simulink model "HW4Prob2"  (R2021a)
settings: Solver=VariableStepAuto  StartTime=0.0  StopTime=10.0  RelTol=1e-3
model workspace (MAT data in the model file):
  L = 1
  theta_dot = 1
  v = 1
  vL = 1
  vR = 1
  w = 1
undefined symbols (not defined in the file): IC, kh, kv, p
settings Model: Creator=Jacob  LastModifiedBy=Jacob

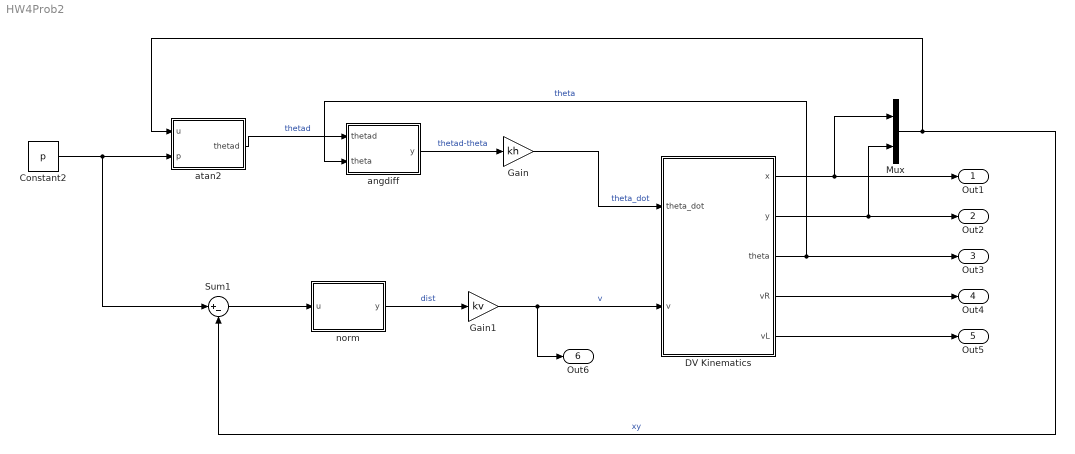
== system HW4Prob2 ==
  Constant2 : Constant  Value=p  VectorParams1D=off
  DV Kinematics : Subsystem
  Gain : Gain  Gain=kh
  Gain1 : Gain  Gain=kv
  Mux : Mux  Inputs=2
  Sum1 : Sum  Inputs=|+-
  angdiff : MATLAB Function  TreatAsAtomicUnit=on
  atan2 : MATLAB Function  TreatAsAtomicUnit=on
  norm : MATLAB Function  TreatAsAtomicUnit=on
  Out1 : Outport  SignalName=x
  Out2 : Outport  Port=2  SignalName=y
  Out3 : Outport  Port=3  SignalName=theta
  Out4 : Outport  Port=4  SignalName=vR
  Out5 : Outport  Port=5  SignalName=vL
  Out6 : Outport  Port=6  SignalName=v
  wires:
  Gain/1 -> DV Kinematics/1(theta_dot)  "theta_dot"
  Gain1/1 -> Out6/1, DV Kinematics/2(v)  "v"
  DV Kinematics/1(x) -> Mux/1, Out1/1
  DV Kinematics/2(y) -> Mux/2, Out2/1
  DV Kinematics/3(theta) -> Out3/1, angdiff/2(theta)  "theta"
  DV Kinematics/4(vR) -> Out4/1
  DV Kinematics/5(vL) -> Out5/1
  Mux/1 -> atan2/1(u), Sum1/2  "xy"
  Constant2/1 -> Sum1/1, atan2/2(p)
  Sum1/1 -> norm/1(u)
  norm/1(y) -> Gain1/1  "dist"
  angdiff/1(y) -> Gain/1  "thetad-theta"
  atan2/1(thetad) -> angdiff/1(thetad)  "thetad"

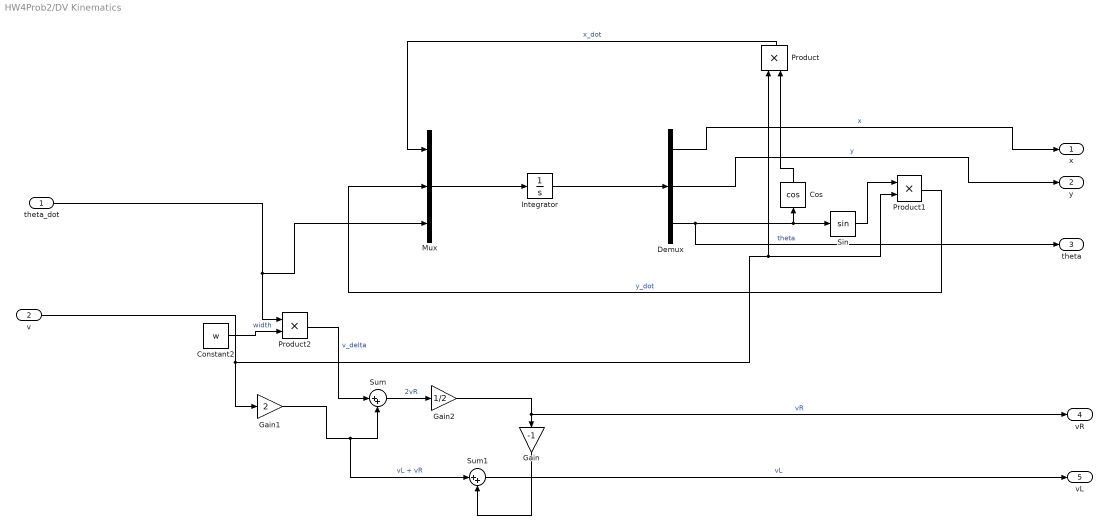
== system HW4Prob2/DV Kinematics ==
  theta_dot : Inport
  v : Inport  Port=2
  Constant2 : Constant  Value=w
  Cos : Trigonometry  Operator=cos
  Demux : Demux  Outputs=3
  Gain : Gain  Gain=-1
  Gain1 : Gain  Gain=2
  Gain2 : Gain  Gain=1/2
  Integrator : Integrator  InitialCondition=IC
  Mux : Mux  Inputs=3
  Product : Product
  Product1 : Product
  Product2 : Product
  Sin : Trigonometry
  Sum : Sum  Inputs=|++
  Sum1 : Sum  Inputs=|++
  x : Outport
  y : Outport  Port=2
  theta : Outport  Port=3
  vR : Outport  Port=4
  vL : Outport  Port=5
  wires:
  Product/1 -> Mux/1  "x_dot"
  Integrator/1 -> Demux/1
  Product1/1 -> Mux/2  "y_dot"
  Constant2/1 -> Product2/2  "width"
  Gain1/1 -> Sum1/1, Sum/2  "vL + vR"
  Demux/3 -> theta/1, Cos/1, Sin/1  "theta"
  v/1 -> Gain1/1, Product1/2, Product/1
  theta_dot/1 -> Product2/1, Mux/3
  Gain2/1 -> vR/1, Gain/1  "vR"
  Sin/1 -> Product1/1
  Cos/1 -> Product/2
  Mux/1 -> Integrator/1
  Sum/1 -> Gain2/1  "2vR"
  Product2/1 -> Sum/1  "v_delta"
  Gain/1 -> Sum1/2
  Demux/1 -> x/1  "x"
  Demux/2 -> y/1  "y"
  Sum1/1 -> vL/1  "vL"

== matlab function HW4Prob2/atan2 ==
  data: u input; thetad output; p input
function thetad = fcn(u,p)

thetad = atan2(p(2)-u(2),p(1)-u(1));

== matlab function HW4Prob2/angdiff ==
  data: thetad input; theta input; y output
function y = fcn(thetad,theta)

y = angdiff(thetad,theta);

== matlab function HW4Prob2/norm ==
  data: u input; y output
function y = fcn(u)

y = norm(u);
